simulink model "model_step_input"  (R2021a)
settings: Solver=ode4  StartTime=0.0  StopTime=STOP  FixedStep=tau  MaxStep=0.001  MinStep=0.0001  RelTol=1e-3
undefined symbols (not defined in the file): a, b, c, d, I, tau
settings Model: Creator=feder  LastModifiedBy=giuseppe
settings SolverCC: AlgebraicLoopSolver=LineSearch
settings DebuggingCC: SFMachineParentedDataDiag=warning

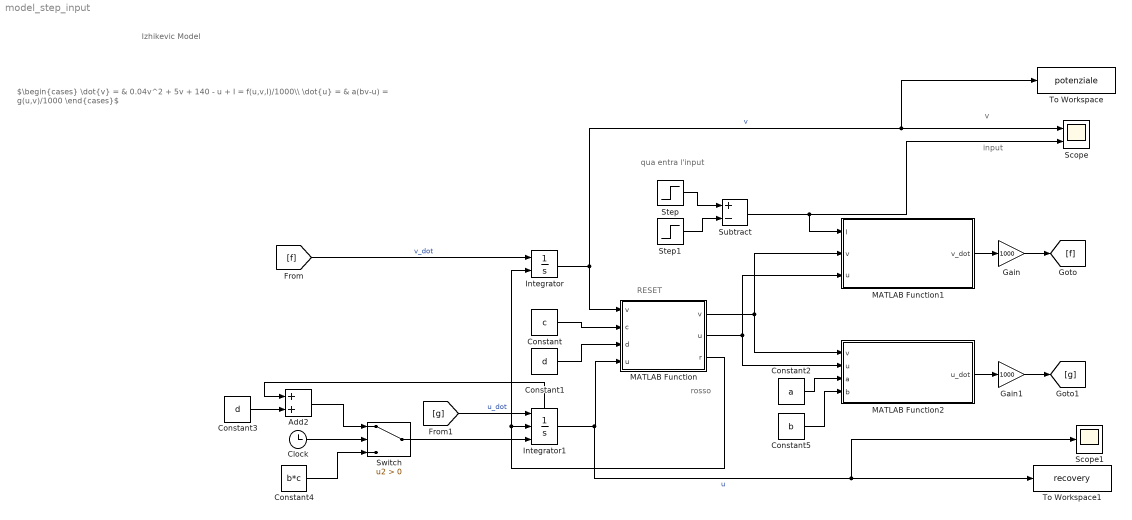
== system model_step_input ==
  note: rosso
  note: input
  note: v
  note: qua entra l'input
  note: RESET
  note: Izhikevic Model
  note: $\begin{cases} \dot{v} = & 0.04v^2 + 5v + 140 - u + I = f(u,v,I)/1000\\ \dot{u} = & a(bv-u) = g(u,v)/1000 \end{cases}$
  Add2 : Sum
  Clock : Clock
  Constant : Constant  Value=c
  Constant1 : Constant  Value=d
  Constant2 : Constant  Value=a
  Constant3 : Constant  Value=d
  Constant4 : Constant  Value=b*c
  Constant5 : Constant  Value=b
  Gain : Gain  Gain=1000
  Gain1 : Gain  Gain=1000
  Integrator : Integrator  ExternalReset=rising  InitialCondition=c  LimitOutput=on  UpperSaturationLimit=30
  Integrator1 : Integrator  ExternalReset=rising  InitialConditionSource=external  InitialCondition=d  ShowStatePort=on
  MATLAB Function : MATLAB Function  TreatAsAtomicUnit=on
  MATLAB Function1 : MATLAB Function  TreatAsAtomicUnit=on
  MATLAB Function2 : MATLAB Function  TreatAsAtomicUnit=on
  Scope : Scope  NumInputPorts=2
  Scope1 : Scope
  Step : Step  Time=round(0.1/tau)*tau  After=I  SampleTime=0
  Step1 : Step  Time=round(0.45/tau)*tau  After=I  SampleTime=0
  Subtract : Sum  Inputs=+-
  Switch : Switch  Criteria=u2 > Threshold
  To Workspace : ToWorkspace  VariableName=potenziale  SaveFormat=Timeseries  SampleTime=-1
  To Workspace1 : ToWorkspace  VariableName=recovery  SaveFormat=Timeseries  SampleTime=-1
  wires:
  Integrator/1 -> MATLAB Function/1("v "), To Workspace/1, Scope/1  "v"
  [f] -> Integrator/1  "v_dot"
  [g] -> Integrator1/1  "u_dot"
  MATLAB Function2/1(u_dot) -> Gain1/1
  Constant/1 -> MATLAB Function/2(c)
  Constant1/1 -> MATLAB Function/3(d)
  Integrator1/1 -> Scope1/1, To Workspace1/1, MATLAB Function/4("u ")  "u"
  MATLAB Function/1(v) -> MATLAB Function2/1(v), MATLAB Function1/2(v)
  MATLAB Function/3(r) -> Integrator/2, Integrator1/2
  Constant3/1 -> Add2/2
  Integrator1/State -> Add2/1
  Switch/1 -> Integrator1/3
  Add2/1 -> Switch/1
  Clock/1 -> Switch/2
  Constant4/1 -> Switch/3
  MATLAB Function1/1(v_dot) -> Gain/1
  MATLAB Function/2(u) -> MATLAB Function2/2(u), MATLAB Function1/3(u)
  Constant2/1 -> MATLAB Function2/3(a)
  Constant5/1 -> MATLAB Function2/4(b)
  Gain/1 -> [f]
  Gain1/1 -> [g]
  Step/1 -> Subtract/1
  Step1/1 -> Subtract/2
  Subtract/1 -> MATLAB Function1/1(I), Scope/2

== matlab function model_step_input/MATLAB Function1 ==
  data: I input; v input; u input; v_dot output
function v_dot = f(I,v,u)

v_dot = 0.04*v^2 + 5*v + 140 + I - u;

end

== matlab function model_step_input/MATLAB Function ==
  data: v input; c input; d input; u input; v output; u output; r output
function [v, u, r] = fcn(v,c,d,u)

if v >= 30
    v = c;
    u = c+d;
    r = 1;
else
    r = 0;
end

== matlab function model_step_input/MATLAB Function2 ==
  data: v input; u input; u_dot output; a input; b input
function u_dot = g(v,u,a,b)

u_dot = a*(b*v-u);

end
